simulink model "three_bus_current_inj_bal"  (R2024b)
settings: Solver=VariableStepAuto  StartTime=0.0  StopTime=1  RelTol=1e-3
libraries: spsACCurrentSourceLib x3, spsGroundLib x3, spsLoadFlowBusLib x3, spsThreePhasePISectionLineLib x3, spsThreePhaseVIMeasurementLib x3, spsThreePhaseSourceLib x2, spsThreePhaseParallelRLCLoadLib x1, spspowerguiLib x1
settings Model: Creator=User  LastModifiedBy=alexapf.stu
settings ModelReferenceCC: EnableRefExpFcnMdlSchedulingChecks=on
settings RTWCC: GPUComputeCapability=3.5  DLArmComputeVersion=19.05

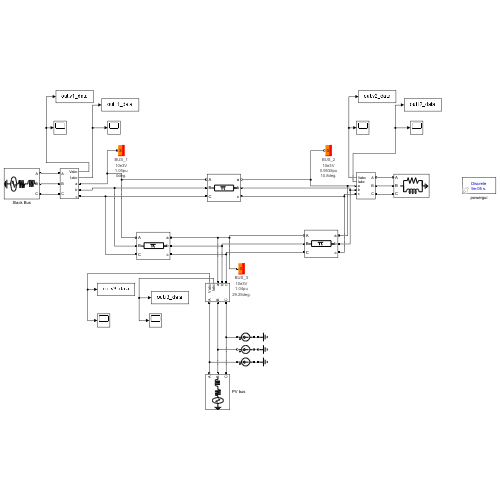
[thumbnail: Simulink's stored preview of the top-level diagram]
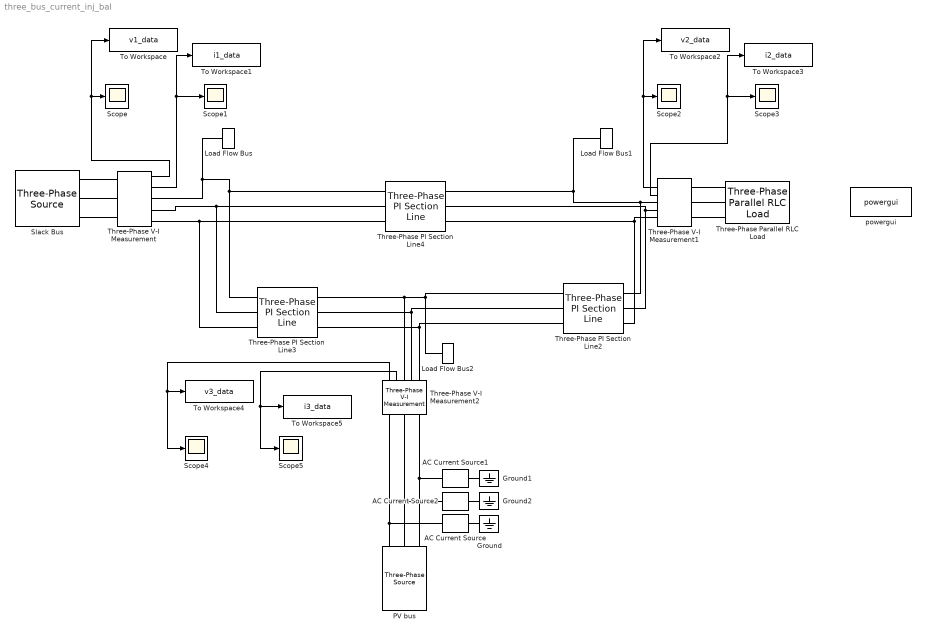
== system three_bus_current_inj_bal ==
  AC Current Source : spsACCurrentSourceLib/AC Current Source  Amplitude=160  Phase=0  Frequency=63  SampleTime=0  Measurements=None
      settings: LibrarySourceBlock=sps_lib/Sources/AC Current Source
  AC Current Source1 : spsACCurrentSourceLib/AC Current Source  Amplitude=160  Phase=120  Frequency=63  SampleTime=0  Measurements=None
      settings: LibrarySourceBlock=sps_lib/Sources/AC Current Source
  AC Current Source2 : spsACCurrentSourceLib/AC Current Source  Amplitude=160  Phase=-120  Frequency=63  SampleTime=0  Measurements=None
      settings: LibrarySourceBlock=sps_lib/Sources/AC Current Source
  Ground : spsGroundLib/Ground  LConnTagsString=a
  Ground1 : spsGroundLib/Ground  LConnTagsString=a
  Ground2 : spsGroundLib/Ground  LConnTagsString=a
  Load Flow Bus : spsLoadFlowBusLib/Load Flow Bus  LConnTagsString=a  Phases=single  Connectors=on one side  ID=BUS_1  Vbase=10e3  Vref=1.05  Vangle=0  VLF=1.05  VLFb=1  VLFc=1  angleLF=0  angleLFb=0  angleLFc=0
  Load Flow Bus1 : spsLoadFlowBusLib/Load Flow Bus  LConnTagsString=a  Phases=single  Connectors=on one side  ID=BUS_2  Vbase=10e3  Vref=1  Vangle=0  VLF=0.9538  VLFb=1  VLFc=1  angleLF=10.8  angleLFb=0  angleLFc=0
  Load Flow Bus2 : spsLoadFlowBusLib/Load Flow Bus  LConnTagsString=a  Phases=single  Connectors=on one side  ID=BUS_3  Vbase=10e3  Vref=1.04  Vangle=0  VLF=1.04  VLFb=1  VLFc=1  angleLF=29.25  angleLFb=0  angleLFc=0
  PV bus : spsThreePhaseSourceLib/Three-Phase Source  InternalConnection=Yg  VoltagePhases=off  Voltage=10e3  PhaseAngle=0  Voltage_phases=[25e3 25e3 25e3]/sqrt(3)  PhaseAngles_phases=[0 -120 +120]  Frequency=60  NonIdealSource=on  SpecifyImpedance=on  Resistance=1e-6  Inductance=1e-6  ShortCircuitLevel=100e6  BaseVoltage=10e3  XRratio=100000  BusType=PV  Pref=200000000  Qref=0  Prefabc=[10e3, 10e3, 10e3]  Qrefabc=[0, 0, 0]  Qmin=-Inf  Qmax=Inf
  Scope{,1..5} (6 alike) : Scope
  Slack Bus : spsThreePhaseSourceLib/Three-Phase Source  InternalConnection=Yg  VoltagePhases=off  Voltage=10e3  PhaseAngle=0  Voltage_phases=[25e3 25e3 25e3]/sqrt(3)  PhaseAngles_phases=[0 -120 +120]  Frequency=60  NonIdealSource=on  SpecifyImpedance=on  Resistance=1e-6  Inductance=1e-6  ShortCircuitLevel=100e6  BaseVoltage=10e3  XRratio=100000  BusType=swing  Pref=10000  Qref=0  Prefabc=[10e3, 10e3, 10e3]  Qrefabc=[0, 0, 0]  Qmin=-Inf  Qmax=Inf
  Three-Phase PI Section Line2 : spsThreePhasePISectionLineLib/Three-Phase PI Section Line  LConnTagsString=a|b|c  RConnTagsString=A|B|C  Length=1  Frequency=60  Resistances=[0.2 0.02]  Inductances=[1.61/(2*pi*50) 5e-4]  Capacitances=[0.0153/(2*pi*50) 2e-8]
  Three-Phase PI Section Line3 : spsThreePhasePISectionLineLib/Three-Phase PI Section Line  LConnTagsString=a|b|c  RConnTagsString=A|B|C  Length=1  Frequency=60  Resistances=[0.1 0.02]  Inductances=[0.92/(2*pi*50) 5e-4]  Capacitances=[0.0079/(2*pi*50) 2e-8]
  Three-Phase PI Section Line4 : spsThreePhasePISectionLineLib/Three-Phase PI Section Line  LConnTagsString=a|b|c  RConnTagsString=A|B|C  Length=1  Frequency=60  Resistances=[0.1/2 0.02]  Inductances=[0.85/(4*pi*50) 5e-4]  Capacitances=[0.0088/(2*pi*50) 2e-8]
  Three-Phase Parallel RLC Load : spsThreePhaseParallelRLCLoadLib/Three-Phase Parallel RLC Load  LConnTagsString=A|B|C  Configuration=Y (grounded)  NominalVoltage=(10000)*0.953767  Vabc=[1e3 1e3 1e3]  Vabcp=[1e3 1e3 1e3]  NominalFrequency=60  UnbalancedPower=off  ActivePower=90000000  InductivePower=30000000  CapacitivePower=0  Pabc=[10e3 9e3 11e3]  QLabc=[100 90 110]  QCabc=[100 90 110]  Pabcp=[10e3 9e3 11e3]  QLabcp=[100 90 110]  QCabcp=[100 90 110]  Measurements=None  LoadType=constant Z
  Three-Phase V-I Measurement : spsThreePhaseVIMeasurementLib/Three-Phase V-I Measurement  VoltageMeasurement=phase-to-ground  SetLabelV=off  LabelV=Vabc  Vpu=on  VpuLL=off  CurrentMeasurement=yes  SetLabelI=off  LabelI=Iabc  Ipu=on  Pbase=10e6  Vbase=10e3  OutputType=Complex  PhasorSimulation=off  PSBequivalent=0
  Three-Phase V-I Measurement1 : spsThreePhaseVIMeasurementLib/Three-Phase V-I Measurement  VoltageMeasurement=phase-to-ground  SetLabelV=off  LabelV=Vabc  Vpu=on  VpuLL=off  CurrentMeasurement=yes  SetLabelI=off  LabelI=Iabc  Ipu=on  Pbase=10e6  Vbase=10e3  OutputType=Complex  PhasorSimulation=off  PSBequivalent=0
  Three-Phase V-I Measurement2 : spsThreePhaseVIMeasurementLib/Three-Phase V-I Measurement  VoltageMeasurement=phase-to-ground  SetLabelV=off  LabelV=Vabc  Vpu=on  VpuLL=off  CurrentMeasurement=yes  SetLabelI=off  LabelI=Iabc  Ipu=on  Pbase=10e6  Vbase=10e3  OutputType=Complex  PhasorSimulation=off  PSBequivalent=0
  To Workspace : ToWorkspace  VariableName=v1_data  SampleTime=-1
  To Workspace1 : ToWorkspace  VariableName=i1_data  SampleTime=-1
  To Workspace2 : ToWorkspace  VariableName=v2_data  SampleTime=-1
  To Workspace3 : ToWorkspace  VariableName=i2_data  SampleTime=-1
  To Workspace4 : ToWorkspace  VariableName=v3_data  SampleTime=-1
  To Workspace5 : ToWorkspace  VariableName=i3_data  SampleTime=-1
  powergui : spspowerguiLib/powergui  Priority=1  SimulationMode=Discrete  SampleTime=50e-6  frequency=60  Iterations=50  frequencyindice=60  Pbase=100e6  ErrMax=1e-4  UnitsV=kV  UnitsW=MW  buscounter=0  FunctionMessages=off  echomessages=off  EnableUseOfTLC=off  CurrentSourceSwitches=off  DisableSnubberDevices=off  DisableRonSwitches=off  DisableVfSwitches=off  DisplayEquations=off  AutomaticDiscreteSolvers=off  SolverType=Tustin/Backward Euler (TBE)  Interpol=off  ExternalGateDelay=off  methode=off  Ts=100  x0status=blocks  SPID=on  SwTol=0  HookPort=off  NonlinearTolerance=1e-4  nMaxIteration=100  ContinueOnMaxIteration=off  RestoreLinks=warning  ResistiveCurrentMeasurement=off  Frange=[0:2:500]  Ylog=off  Xlog=on  ShowGrid=off  save=off  variable=ZData  structure=0  ZoomFFT=off  StartTime=0.0  cycles=1  DisplayStyle=1  fundamental=60  FreqAxis=off  MaxFrequency=1000  frequencyindicesteady=1  RmsSteady=1  display=off
  wires:
  Three-Phase V-I Measurement/1 -> Scope/1, To Workspace/1
  Three-Phase V-I Measurement/2 -> To Workspace1/1, Scope1/1
  Three-Phase V-I Measurement1/1 -> Scope2/1, To Workspace2/1
  Three-Phase V-I Measurement1/2 -> To Workspace3/1, Scope3/1
  Three-Phase V-I Measurement2/1 -> Scope4/1, To Workspace4/1
  Three-Phase V-I Measurement2/2 -> Scope5/1, To Workspace5/1
  connections:
  Slack Bus/RConn3 -- Three-Phase V-I Measurement/LConn3
  Slack Bus/RConn2 -- Three-Phase V-I Measurement/LConn2
  Slack Bus/RConn1 -- Three-Phase V-I Measurement/LConn1
  Three-Phase V-I Measurement1/RConn1 -- Three-Phase PI Section Line4/RConn1 -- Load Flow Bus1/LConn1 -- Three-Phase PI Section Line2/RConn1
  Three-Phase PI Section Line4/RConn2 -- Three-Phase PI Section Line2/RConn2 -- Three-Phase V-I Measurement1/RConn2
  Three-Phase PI Section Line4/RConn3 -- Three-Phase V-I Measurement1/RConn3 -- Three-Phase PI Section Line2/RConn3
  PV bus/RConn1 -- Three-Phase V-I Measurement2/LConn1 -- AC Current Source/RConn1
  PV bus/RConn2 -- AC Current Source2/RConn1 -- Three-Phase V-I Measurement2/LConn2
  PV bus/RConn3 -- AC Current Source1/RConn1 -- Three-Phase V-I Measurement2/LConn3
  Three-Phase V-I Measurement1/LConn1 -- Three-Phase Parallel RLC Load/LConn1
  Three-Phase V-I Measurement1/LConn2 -- Three-Phase Parallel RLC Load/LConn2
  Three-Phase V-I Measurement1/LConn3 -- Three-Phase Parallel RLC Load/LConn3
  Load Flow Bus/LConn1 -- Three-Phase PI Section Line4/LConn1 -- Three-Phase PI Section Line3/LConn1 -- Three-Phase V-I Measurement/RConn1
  Three-Phase V-I Measurement/RConn2 -- Three-Phase PI Section Line4/LConn2 -- Three-Phase PI Section Line3/LConn2
  Three-Phase V-I Measurement/RConn3 -- Three-Phase PI Section Line4/LConn3 -- Three-Phase PI Section Line3/LConn3
  Three-Phase PI Section Line3/RConn1 -- Three-Phase PI Section Line2/LConn1 -- Load Flow Bus2/LConn1 -- Three-Phase V-I Measurement2/RConn1
  Three-Phase PI Section Line3/RConn2 -- Three-Phase PI Section Line2/LConn2 -- Three-Phase V-I Measurement2/RConn2
  Three-Phase PI Section Line3/RConn3 -- Three-Phase PI Section Line2/LConn3 -- Three-Phase V-I Measurement2/RConn3
  AC Current Source/LConn1 -- Ground/LConn1
  AC Current Source1/LConn1 -- Ground1/LConn1
  AC Current Source2/LConn1 -- Ground2/LConn1
